simulink model "motor_model_twoPole"  (R2017a)
settings: Solver=ode45  StartTime=0.0  StopTime=150  RelTol=1e-3  EnableMultiTasking=on
values from neighbouring files (symbols this model uses):
  B = 0.21e-05    (= 2.1e-06)    [parameters.m]
  I = Irt+Iw    (= 3.06520589874e-05)    [parameters.m]
  KM = 0.0065    [parameters.m]
  Kv = KM    (= 0.0065)    [parameters.m]
  rad2rpm = 60/(2*pi)    (= 9.54929658551)    [parameters.m]
libraries: simulink x1
settings Model: Creator=root  LastModifiedBy=hernan
settings DataIOCC: LimitDataPoints=on  SaveFormat=Array  SignalLoggingSaveFormat=ModelDataLogs
settings OptimizationCC: ExpressionDepthLimit=2147483647  LifeSpan=inf
settings DebuggingCC: UnderspecifiedInitializationDetection=Classic  MergeDetectMultiDrivingBlocksExec=none  SolverPrmCheckMsg=warning  FcnCallInpInsideContextMsg=warning  StateNameClashWarn=warning  SFUnexpectedBacktrackingDiag=warning  SFNoUnconditionalDefaultTransitionDiag=warning  SFExecutionAtInitializationDiag=none
settings HardwareCC: ProdBitPerPointer=32  ProdBitPerSizeT=32  ProdBitPerPtrDiffT=32  ProdLargestAtomicFloat=None  ProdIntDivRoundTo=Undefined  ProdEndianess=Unspecified  ProdWordSize=32  ProdHWDeviceType=32-bit Generic
settings ModelReferenceCC: PropagateSignalLabelsOutOfModel=off
settings GRTTargetCC: TargetLangStandard=C89/C90 (ANSI)  GeneratePreprocessorConditionals=Disable all
settings ConfigComp: CovMetricSettings=dw  CovHtmlReporting=on  CovSaveCumulativeToWorkspaceVar=on  CovSaveSingleToWorkspaceVar=on  CovExternalEMLEnable=off

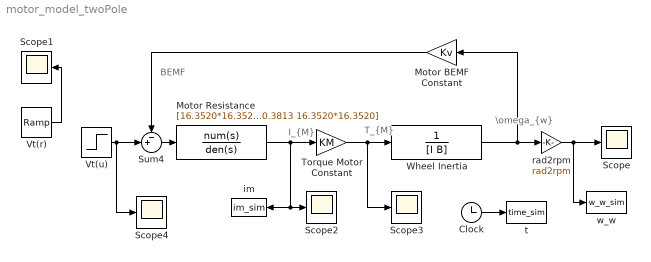
== system motor_model_twoPole ==
  note: T_{M}
  note: I_{M}
  note: BEMF
  note: \omega_{w}
  Clock : Clock
  Motor BEMF Constant : Gain  Gain=Kv
  Motor Resistance : TransferFcn  Numerator=[16.3520*16.3520]  Denominator=[1 2*16.3520*0.3813 16.3520*16.3520]
  Scope{,1..4} (5 alike) : Scope
  Sum4 : Sum  Inputs=-+|
  Torque Motor Constant : Gain  Gain=KM
  Vt(r) : simulink/Sources/Ramp  slope=1  start=0  X0=0
  Vt(u) : Step  After=2.5  SampleTime=0
  Wheel Inertia : TransferFcn  Denominator=[I B]
  im : ToWorkspace  VariableName=im_sim  SampleTime=-1
      settings: Save2DSignal=2-D array (concatenate along first dimension)
  rad2rpm : Gain  Gain=rad2rpm
  t : ToWorkspace  VariableName=time_sim  SampleTime=-1
      settings: Save2DSignal=2-D array (concatenate along first dimension)
  w_w : ToWorkspace  VariableName=w_w_sim  SampleTime=-1
      settings: Save2DSignal=2-D array (concatenate along first dimension)
  wires:
  Sum4/1 -> Motor Resistance/1
  Motor Resistance/1 -> Torque Motor Constant/1, im/1, Scope2/1
  Torque Motor Constant/1 -> Wheel Inertia/1, Scope3/1
  Motor BEMF Constant/1 -> Sum4/1
  Vt(r)/1 -> Scope1/1
  Vt(u)/1 -> Sum4/2, Scope4/1
  Wheel Inertia/1 -> rad2rpm/1, Motor BEMF Constant/1
  rad2rpm/1 -> w_w/1, Scope/1
  Clock/1 -> t/1
